simulink model "profacc_sim"  (R2025b)
settings: Solver=ode45  StartTime=0.0  StopTime=40.0  RelTol=1e-3
settings Model: Creator=sprinkle  LastModifiedBy=sprinkle
settings OptimizationCC: ReuseModelBlockBuffer=off
settings RTWCC: GPUComputeCapability=3.5

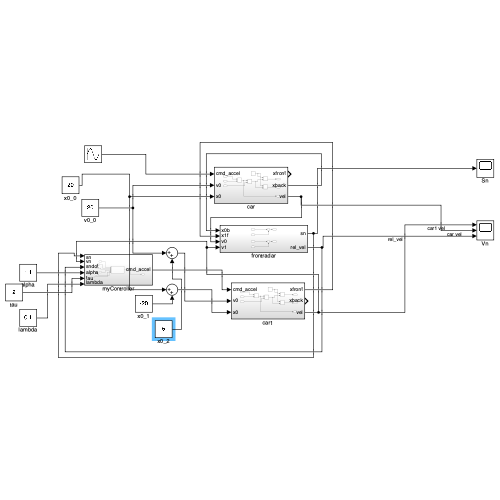
[thumbnail: Simulink's stored preview of the top-level diagram]
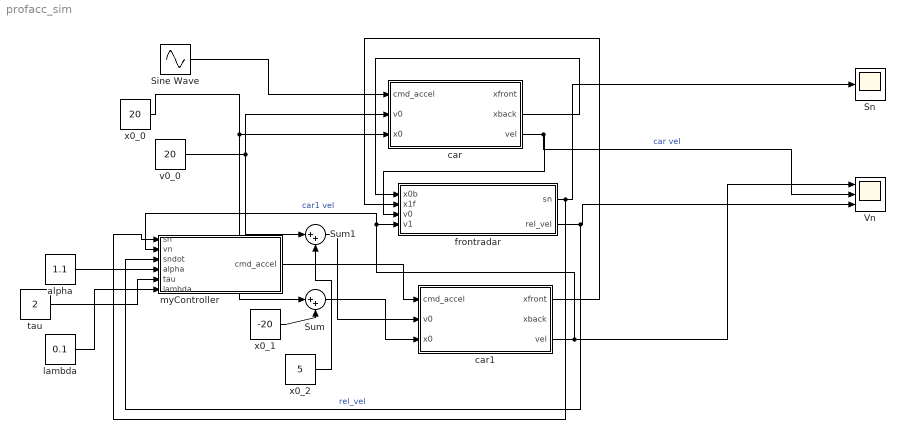
== system profacc_sim ==
  Sine Wave : Sin  Amplitude=0.5  SampleTime=0
  Sn : Scope
      settings: ActiveDisplayYMinimum=12.539748013242225  ActiveDisplayYMaximum=44.742267880819952
  Sum : Sum  Inputs=|++
  Sum1 : Sum  Inputs=|++
  Vn : Scope  NumInputPorts=3
      settings: ActiveDisplayYMinimum=-15.489718822251529  ActiveDisplayYMaximum=35.697668945320132
  alpha : Constant  Value=1.1
  car : Subsystem
  car1 : Subsystem
  frontradar : Subsystem
  lambda : Constant  Value=0.1
  myController : Subsystem
  tau : Constant  Value=2
  v0_0 : Constant  Value=20
  x0_0 : Constant  Value=20
  x0_1 : Constant  Value=-20
  x0_2 : Constant  Value=5
  wires:
  Sine Wave/1 -> car/1(cmd_accel)
  v0_0/1 -> car/2(v0), Sum1/1
  x0_0/1 -> Sum/1, car/3(x0)
  x0_1/1 -> Sum/2
  Sum/1 -> car1/3(x0)
  x0_2/1 -> Sum1/2
  Sum1/1 -> car1/2(v0)
  car/2(xback) -> frontradar/1(x0b)
  car1/1(xfront) -> frontradar/2(x1f)
  car/3(vel) -> Vn/2, frontradar/3(v0)  "car vel"
  car1/3(vel) -> Vn/1, myController/2(vn), frontradar/4(v1)  "car1 vel"
  frontradar/1(sn) -> myController/1(sn), Sn/1
  frontradar/2(rel_vel) -> myController/3(sndot), Vn/3  "rel_vel"
  alpha/1 -> myController/4(alpha)
  tau/1 -> myController/5(tau)
  myController/1(cmd_accel) -> car1/1(cmd_accel)
  lambda/1 -> myController/6(lambda)

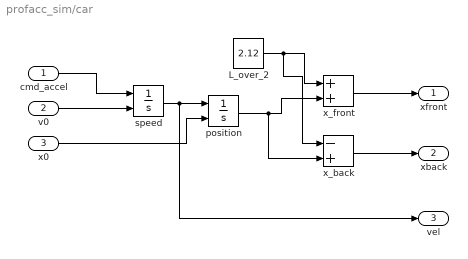
== system profacc_sim/car ==
  cmd_accel : Inport
  v0 : Inport  Port=2
  x0 : Inport  Port=3
  L_over_2 : Constant  Value=2.12
  position : Integrator  InitialConditionSource=external
  speed : Integrator  InitialConditionSource=external
  x_back : Sum  Inputs=-+
  x_front : Sum
  xfront : Outport
  xback : Outport  Port=2
  vel : Outport  Port=3
  wires:
  x_back/1 -> xback/1
  x0/1 -> position/2
  cmd_accel/1 -> speed/1
  speed/1 -> vel/1, position/1
  position/1 -> x_back/2, x_front/2
  x_front/1 -> xfront/1
  v0/1 -> speed/2
  L_over_2/1 -> x_back/1, x_front/1

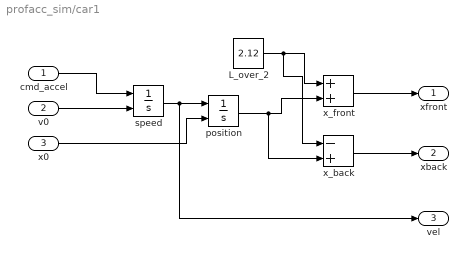
== system profacc_sim/car1 ==
  cmd_accel : Inport
  v0 : Inport  Port=2
  x0 : Inport  Port=3
  L_over_2 : Constant  Value=2.12
  position : Integrator  InitialConditionSource=external
  speed : Integrator  InitialConditionSource=external
  x_back : Sum  Inputs=-+
  x_front : Sum
  xfront : Outport
  xback : Outport  Port=2
  vel : Outport  Port=3
  wires:
  x_back/1 -> xback/1
  x0/1 -> position/2
  cmd_accel/1 -> speed/1
  speed/1 -> vel/1, position/1
  position/1 -> x_back/2, x_front/2
  x_front/1 -> xfront/1
  v0/1 -> speed/2
  L_over_2/1 -> x_back/1, x_front/1

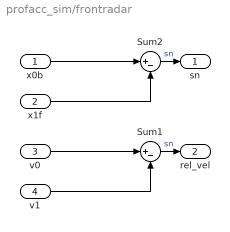
== system profacc_sim/frontradar ==
  x0b : Inport
  x1f : Inport  Port=2
  v0 : Inport  Port=3
  v1 : Inport  Port=4
  Sum1 : Sum  Inputs=|+-
  Sum2 : Sum  Inputs=|+-
  sn : Outport
  rel_vel : Outport  Port=2
  wires:
  x1f/1 -> Sum2/2
  Sum2/1 -> sn/1  "sn"
  x0b/1 -> Sum2/1
  v0/1 -> Sum1/1
  Sum1/1 -> rel_vel/1  "sn"
  v1/1 -> Sum1/2

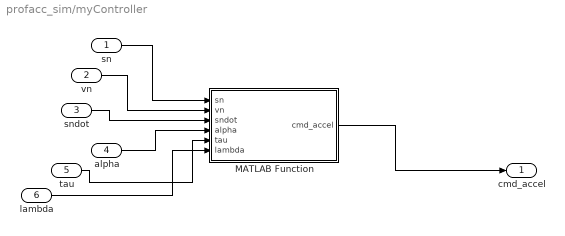
== system profacc_sim/myController ==
  sn : Inport
  vn : Inport  Port=2
  sndot : Inport  Port=3
  alpha : Inport  Port=4
  tau : Inport  Port=5
  lambda : Inport  Port=6
  MATLAB Function : MATLAB Function  TreatAsAtomicUnit=on
  cmd_accel : Outport
  wires:
  MATLAB Function/1(cmd_accel) -> cmd_accel/1
  tau/1 -> MATLAB Function/5(tau)
  alpha/1 -> MATLAB Function/4(alpha)
  sn/1 -> MATLAB Function/1(sn)
  vn/1 -> MATLAB Function/2(vn)
  sndot/1 -> MATLAB Function/3(sndot)
  lambda/1 -> MATLAB Function/6(lambda)

== matlab function profacc_sim/myController/MATLAB Function ==
  data: sn input; cmd_accel output; vn input; sndot input; alpha input; tau input; lambda input
function cmd_accel = fcn(sn,vn,sndot,alpha,tau,lambda)

cmd_accel = alpha * (sn - tau*vn + lambda*sndot);
